simulink model "simulink_robo"  (R2014a)
settings: Solver=ode4  StartTime=0.0  StopTime=Tsim  RelTol=1e-3
values from neighbouring files (symbols this model uses):
  b = 0.1    [simula_robo.m]    (also in simula_robo_thiago.m)
  g = 40    [simula_robo.m]    (also in simula_robo_thiago.m)
  J = 0.01    [simula_robo.m]    (also in simula_robo_thiago.m)
  Kd = 0    [simula_robo.m]    (also in simula_robo_thiago.m)
  Ke = 0.08    [simula_robo.m]    (also in simula_robo_thiago.m)
  Ki = 10.0    (= 10)    [simula_robo.m]    (also in simula_robo_thiago.m = 0)
  Kp = 5.0    (= 5)    [simula_robo.m]    (also in simula_robo_thiago.m = 50)
  ksi = 0.3    [simula_robo.m]    (also in simula_robo_thiago.m)
  L = 0.5    [simula_robo.m]    (also in simula_robo_thiago.m)
  R = 1    [simula_robo.m]    (also in simula_robo_thiago.m)
  thetao = 0.0    (= 0)    [simula_robo.m]    (also in simula_robo_thiago.m)
  Ts = 0.1    [simula_robo.m]    (also in simula_robo_thiago.m)
  xo = 0.0    (= 0)    [simula_robo.m]    (also in simula_robo_thiago.m)
  yo = -0.3    [simula_robo.m]    (also in simula_robo_thiago.m)
libraries: simulink x2, simulink_extras x2
settings Model: Creator=Fabricio  LastModifiedBy=Thiago Lobo
settings DebuggingCC: UnderspecifiedInitializationDetection=Classic  StateNameClashWarn=warning

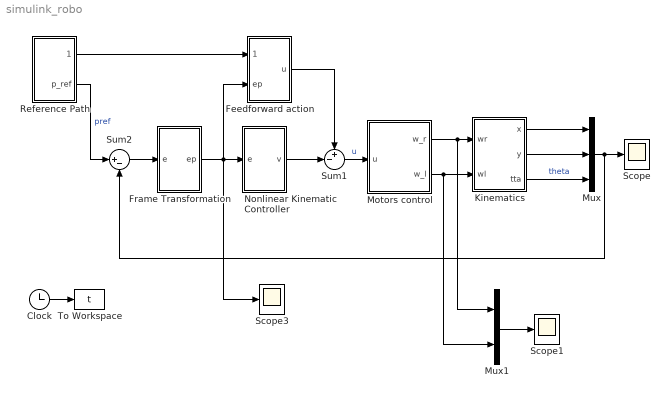
== system simulink_robo ==
  Clock : Clock
  Feedforward action : Subsystem
  Frame Transformation : Subsystem
  Kinematics : Subsystem
  Motors control : Subsystem
  Mux : Mux  Inputs=3
  Mux1 : Mux  Inputs=2
  Nonlinear Kinematic Controller : Subsystem
  Reference Path : Subsystem
  Scope : Scope
      settings: TimeRange=10
  Scope1 : Scope
      settings: TimeRange=10  SaveName=ScopeData2
  Scope3 : Scope
      settings: TimeRange=10  SaveName=ScopeData4
  Sum1 : Sum  Inputs=+-|
  Sum2 : Sum  Inputs=|+-
  To Workspace : ToWorkspace  VariableName=t  SampleTime=Ts
  wires:
  Kinematics/2(y) -> Mux/2
  Kinematics/3(tta) -> Mux/3  "theta"
  Motors control/1(w_r) -> Mux1/1, Kinematics/1(wr)
  Frame Transformation/1(ep) -> Scope3/1, Nonlinear Kinematic Controller/1(e), Feedforward action/2(ep)
  Reference Path/2(p_ref) -> Sum2/1  "pref"
  Reference Path/1(vw_ref) -> Feedforward action/1(vw_ref)
  Sum1/1 -> Motors control/1(u)  "u"
  Clock/1 -> To Workspace/1
  Mux/1 -> Scope/1, Sum2/2
  Sum2/1 -> Frame Transformation/1(e)
  Feedforward action/1(u) -> Sum1/1
  Motors control/2(w_l) -> Mux1/2, Kinematics/2(wl)
  Kinematics/1(x) -> Mux/1
  Nonlinear Kinematic Controller/1(v) -> Sum1/2
  Mux1/1 -> Scope1/1

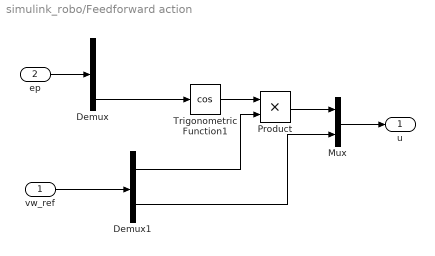
== system simulink_robo/Feedforward action ==
  vw_ref : Inport
  ep : Inport  Port=2
  Demux : Demux  Outputs=3
  Demux1 : Demux  Outputs=2
  Mux : Mux  Inputs=2
  Product : Product
  Trigonometric Function1 : Trigonometry  Operator=cos
  u : Outport
  wires:
  ep/1 -> Demux/1
  vw_ref/1 -> Demux1/1
  Demux/3 -> Trigonometric Function1/1
  Product/1 -> Mux/1
  Mux/1 -> u/1
  Trigonometric Function1/1 -> Product/1
  Demux1/1 -> Product/2
  Demux1/2 -> Mux/2

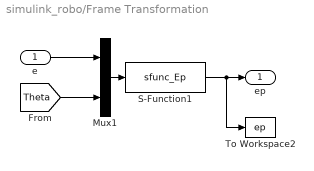
== system simulink_robo/Frame Transformation ==
  e : Inport
  Mux1 : Mux  Inputs=2
  S-Function1 : S-Function  FunctionName=sfunc_Ep  Parameters=Ts  EnableBusSupport=off
  To Workspace2 : ToWorkspace  VariableName=ep  SampleTime=Ts
  ep : Outport
  wires:
  S-Function1/1 -> To Workspace2/1, ep/1
  Mux1/1 -> S-Function1/1
  e/1 -> Mux1/1
  [Theta] -> Mux1/2

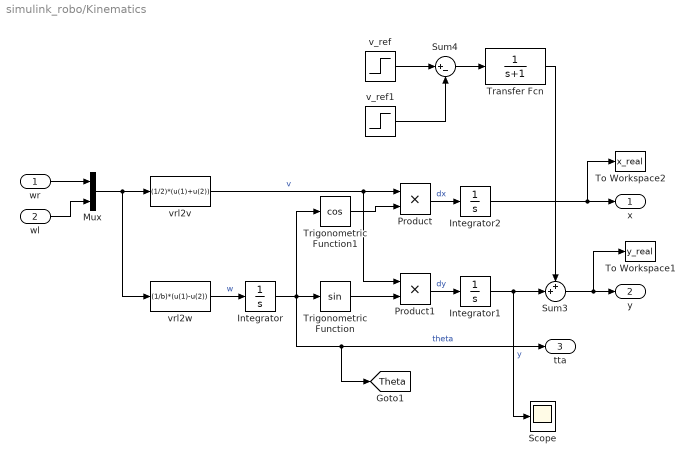
== system simulink_robo/Kinematics ==
  wr : Inport
  wl : Inport  Port=2
  Integrator : Integrator  InitialCondition=thetao
  Integrator1 : Integrator  InitialCondition=yo
  Integrator2 : Integrator  InitialCondition=xo
  Mux : Mux  Inputs=2
  Product : Product
  Product1 : Product
  Scope : Scope
      settings: TimeRange=10
  Sum3 : Sum  Inputs=++|
  Sum4 : Sum  Inputs=|+-
  To Workspace1 : ToWorkspace  VariableName=y_real  SampleTime=Ts
  To Workspace2 : ToWorkspace  VariableName=x_real  SampleTime=Ts
  Transfer Fcn : TransferFcn  Denominator=[1 1]
  Trigonometric Function : Trigonometry
  Trigonometric Function1 : Trigonometry  Operator=cos
  v_ref : Step  Time=25  After=-0.1  SampleTime=0
  v_ref1 : Step  Time=26  After=-0.1  SampleTime=0
  vrl2v : Fcn  Expr=(1/2)*(u(1)+u(2))
  vrl2w : Fcn  Expr=(1/b)*(u(1)-u(2))
  x : Outport
  y : Outport  Port=2
  tta : Outport  Port=3
  tag scope: Theta=global
  wires:
  wr/1 -> Mux/1
  Trigonometric Function1/1 -> Product/2
  Product/1 -> Integrator2/1  "dx"
  Integrator/1 -> [Theta], tta/1, Trigonometric Function1/1, Trigonometric Function/1  "theta"
  Integrator1/1 -> Sum3/2, Scope/1  "y"
  Product1/1 -> Integrator1/1  "dy"
  Trigonometric Function/1 -> Product1/2
  Mux/1 -> vrl2w/1, vrl2v/1
  wl/1 -> Mux/2
  vrl2w/1 -> Integrator/1  "w"
  vrl2v/1 -> Product/1, Product1/1  "v"
  v_ref/1 -> Sum4/1
  v_ref1/1 -> Sum4/2
  Sum4/1 -> Transfer Fcn/1
  Transfer Fcn/1 -> Sum3/1
  Integrator2/1 -> To Workspace2/1, x/1
  Sum3/1 -> To Workspace1/1, y/1

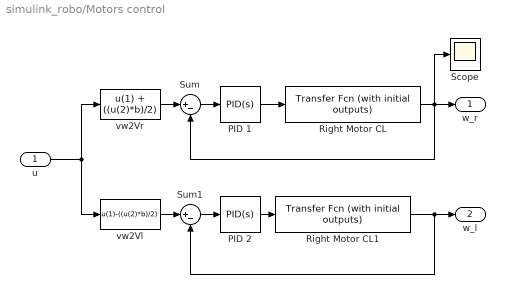
== system simulink_robo/Motors control ==
  u : Inport
  PID 1 : simulink/Continuous/PID Controller  Controller=PID  TimeDomain=Continuous-time  SampleTime=1  IntegratorMethod=Forward Euler  FilterMethod=Forward Euler  Form=Parallel  P=Kp  I=Ki  D=Kd  N=100  InitialConditionSource=internal  InitialConditionForIntegrator=0  InitialConditionForFilter=0  ExternalReset=none  LimitOutput=off  UpperSaturationLimit=inf  LowerSaturationLimit=-inf  LinearizeAsGain=on  AntiWindupMode=none  Kb=1  TrackingMode=off  Kt=1  PParamMin=[]  PParamMax=[]  IParamMin=[]  IParamMax=[]  DParamMin=[]  DParamMax=[]  NParamMin=[]  NParamMax=[]  KbParamMin=[]  KbParamMax=[]  KtParamMin=[]  KtParamMax=[]  POutMin=[]  POutMax=[]  IOutMin=[]  IOutMax=[]  DOutMin=[]  DOutMax=[]  NOutMin=[]  NOutMax=[]  KbOutMin=[]  KbOutMax=[]  KtOutMin=[]  KtOutMax=[]  IntegratorOutMin=[]  IntegratorOutMax=[]  FilterOutMin=[]  FilterOutMax=[]  SumOutMin=[]  SumOutMax=[]  SumI1OutMin=[]  SumI1OutMax=[]  SumI2OutMin=[]  SumI2OutMax=[]  SumI3OutMin=[]  SumI3OutMax=[]  SumDOutMin=[]  SumDOutMax=[]  SaturationOutMin=[]  SaturationOutMax=[]  IntegratorContinuousStateAttributes=''  IntegratorStateMustResolveToSignalObject=off  IntegratorRTWStateStorageClass=Auto  FilterContinuousStateAttributes=''  FilterStateMustResolveToSignalObject=off  FilterRTWStateStorageClass=Auto
  PID 2 : simulink/Continuous/PID Controller  Controller=PID  TimeDomain=Continuous-time  SampleTime=1  IntegratorMethod=Forward Euler  FilterMethod=Forward Euler  Form=Parallel  P=Kp  I=Ki  D=Kd  N=100  InitialConditionSource=internal  InitialConditionForIntegrator=0  InitialConditionForFilter=0  ExternalReset=none  LimitOutput=off  UpperSaturationLimit=inf  LowerSaturationLimit=-inf  LinearizeAsGain=on  AntiWindupMode=none  Kb=1  TrackingMode=off  Kt=1  PParamMin=[]  PParamMax=[]  IParamMin=[]  IParamMax=[]  DParamMin=[]  DParamMax=[]  NParamMin=[]  NParamMax=[]  KbParamMin=[]  KbParamMax=[]  KtParamMin=[]  KtParamMax=[]  POutMin=[]  POutMax=[]  IOutMin=[]  IOutMax=[]  DOutMin=[]  DOutMax=[]  NOutMin=[]  NOutMax=[]  KbOutMin=[]  KbOutMax=[]  KtOutMin=[]  KtOutMax=[]  IntegratorOutMin=[]  IntegratorOutMax=[]  FilterOutMin=[]  FilterOutMax=[]  SumOutMin=[]  SumOutMax=[]  SumI1OutMin=[]  SumI1OutMax=[]  SumI2OutMin=[]  SumI2OutMax=[]  SumI3OutMin=[]  SumI3OutMax=[]  SumDOutMin=[]  SumDOutMax=[]  SaturationOutMin=[]  SaturationOutMax=[]  IntegratorContinuousStateAttributes=''  IntegratorStateMustResolveToSignalObject=off  IntegratorRTWStateStorageClass=Auto  FilterContinuousStateAttributes=''  FilterStateMustResolveToSignalObject=off  FilterRTWStateStorageClass=Auto
  Right Motor CL : simulink_extras/Additional Linear/Transfer Fcn (with initial outputs)  N=[Ke]  D="[J*L  (J*R+b*L) (b*R+Ke^2)]"  Y0=0  U0=0
  Right Motor CL1 : simulink_extras/Additional Linear/Transfer Fcn (with initial outputs)  N=[Ke]  D="[J*L  (J*R+b*L) (b*R+Ke^2)]"  Y0=0  U0=0
  Scope : Scope
      settings: SaveName=ScopeData5
  Sum : Sum  Inputs=|+-
  Sum1 : Sum  Inputs=|+-
  vw2Vl : Fcn  Expr=u(1)-((u(2)*b)/2)
  vw2Vr : Fcn  Expr=u(1) + ((u(2)*b)/2)
  w_r : Outport
  w_l : Outport  Port=2
  wires:
  u/1 -> vw2Vr/1, vw2Vl/1
  Right Motor CL/1 -> Sum/2, Scope/1, w_r/1
  PID 1/1 -> Right Motor CL/1
  Sum/1 -> PID 1/1
  PID 2/1 -> Right Motor CL1/1
  Sum1/1 -> PID 2/1
  vw2Vl/1 -> Sum1/1
  Right Motor CL1/1 -> Sum1/2, w_l/1
  vw2Vr/1 -> Sum/1

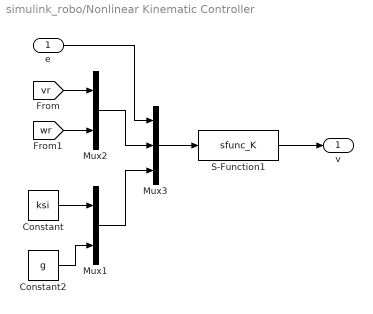
== system simulink_robo/Nonlinear Kinematic Controller ==
  e : Inport
  Constant : Constant  Value=ksi
  Constant2 : Constant  Value=g
  Mux1 : Mux  Inputs=2
  Mux2 : Mux  Inputs=2
  Mux3 : Mux  Inputs=3
  S-Function1 : S-Function  FunctionName=sfunc_K  Parameters=Ts  EnableBusSupport=off
  v : Outport
  wires:
  S-Function1/1 -> v/1
  Constant2/1 -> Mux1/2
  Constant/1 -> Mux1/1
  Mux3/1 -> S-Function1/1
  [vr] -> Mux2/1
  [wr] -> Mux2/2
  Mux2/1 -> Mux3/2
  Mux1/1 -> Mux3/3
  e/1 -> Mux3/1

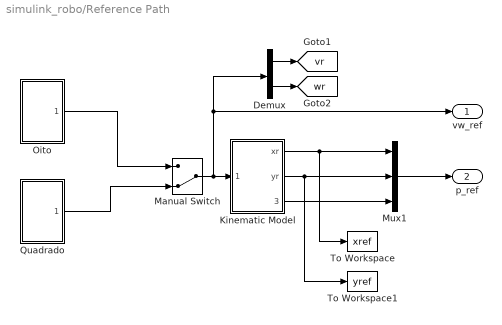
== system simulink_robo/Reference Path ==
  Demux : Demux  Outputs=2
  Kinematic Model : Subsystem
  Manual Switch : ManualSwitch  CurrentSetting=0
  Mux1 : Mux  Inputs=3
  Oito : Subsystem
  Quadrado : Subsystem
  To Workspace : ToWorkspace  VariableName=xref  SampleTime=Ts
  To Workspace1 : ToWorkspace  VariableName=yref  SampleTime=Ts
  vw_ref : Outport
  p_ref : Outport  Port=2
  tag scope: vr=global, wr=global
  wires:
  Kinematic Model/1(xr) -> To Workspace/1, Mux1/1
  Kinematic Model/3(thetar) -> Mux1/3
  Mux1/1 -> p_ref/1
  Kinematic Model/2(yr) -> To Workspace1/1, Mux1/2
  Oito/1(vw_ref) -> Manual Switch/1
  Quadrado/1(vw_ref) -> Manual Switch/2
  Demux/1 -> [vr]
  Demux/2 -> [wr]
  Manual Switch/1 -> vw_ref/1, Demux/1, Kinematic Model/1(vw_ref)

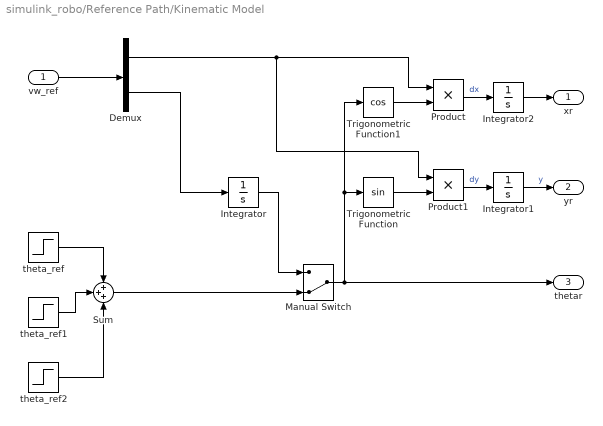
== system simulink_robo/Reference Path/Kinematic Model ==
  vw_ref : Inport
  Demux : Demux  Outputs=2
  Integrator : Integrator
  Integrator1 : Integrator
  Integrator2 : Integrator
  Manual Switch : ManualSwitch  CurrentSetting=0
  Product : Product
  Product1 : Product
  Sum : Sum  Inputs=+++
  Trigonometric Function : Trigonometry
  Trigonometric Function1 : Trigonometry  Operator=cos
  theta_ref : Step  Time=20  After=pi/2  SampleTime=0
  theta_ref1 : Step  Time=40  After=pi/2  SampleTime=0
  theta_ref2 : Step  Time=60  After=pi/2  SampleTime=0
  xr : Outport
  yr : Outport  Port=2
  thetar : Outport  Port=3
  wires:
  Trigonometric Function1/1 -> Product/2
  Product/1 -> Integrator2/1  "dx"
  Integrator/1 -> Manual Switch/1
  Integrator1/1 -> yr/1  "y"
  Product1/1 -> Integrator1/1  "dy"
  Integrator2/1 -> xr/1
  Trigonometric Function/1 -> Product1/2
  Demux/1 -> Product/1, Product1/1
  Demux/2 -> Integrator/1
  vw_ref/1 -> Demux/1
  theta_ref/1 -> Sum/1
  theta_ref1/1 -> Sum/2
  theta_ref2/1 -> Sum/3
  Sum/1 -> Manual Switch/2
  Manual Switch/1 -> Trigonometric Function1/1, Trigonometric Function/1, thetar/1

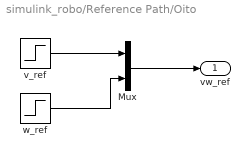
== system simulink_robo/Reference Path/Oito ==
  Mux : Mux  Inputs=2
  v_ref : Step  Before=0.2  After=0.2  SampleTime=0
  w_ref : Step  Time=18  Before=0.35  After=-0.35  SampleTime=0
  vw_ref : Outport
  wires:
  v_ref/1 -> Mux/1
  w_ref/1 -> Mux/2
  Mux/1 -> vw_ref/1

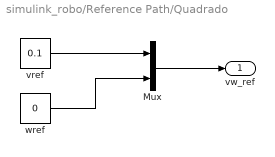
== system simulink_robo/Reference Path/Quadrado ==
  Mux : Mux  Inputs=2
  vref : Constant  Value=0.1
  wref : Constant  Value=0
  vw_ref : Outport
  wires:
  vref/1 -> Mux/1
  wref/1 -> Mux/2
  Mux/1 -> vw_ref/1
